simulink model "dynamic_block"  (R2023b)
settings: Solver=VariableStepAuto  StartTime=0.0  StopTime=10.0  RelTol=1e-3
libraries: matrix_library x1, aerolibutil x1
settings Model: Creator=aryam  LastModifiedBy=aryam

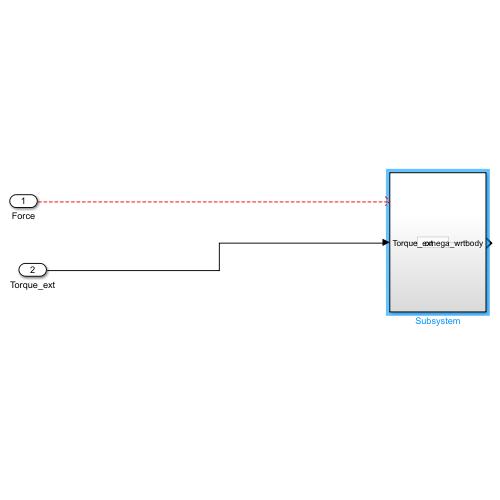
[thumbnail: Simulink's stored preview of the top-level diagram]
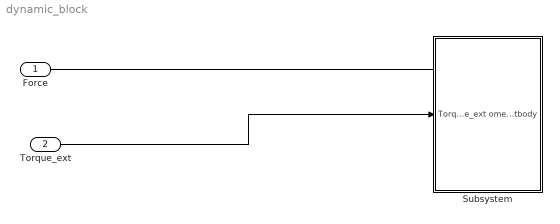
== system dynamic_block ==
  Force : Inport
  Torque_ext : Inport  Port=2  PortDimensions=3
  Subsystem : Subsystem
  wires:
  Force/1 -> ?
  Torque_ext/1 -> Subsystem/1(Torque_ext)

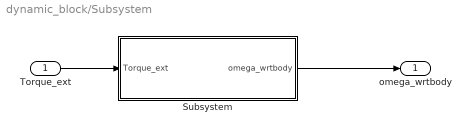
== system dynamic_block/Subsystem ==
  Torque_ext : Inport  PortDimensions=3
  Subsystem : Subsystem
  omega_wrtbody : Outport
  wires:
  Torque_ext/1 -> Subsystem/1(Torque_ext)
  Subsystem/1(omega_wrtbody) -> omega_wrtbody/1

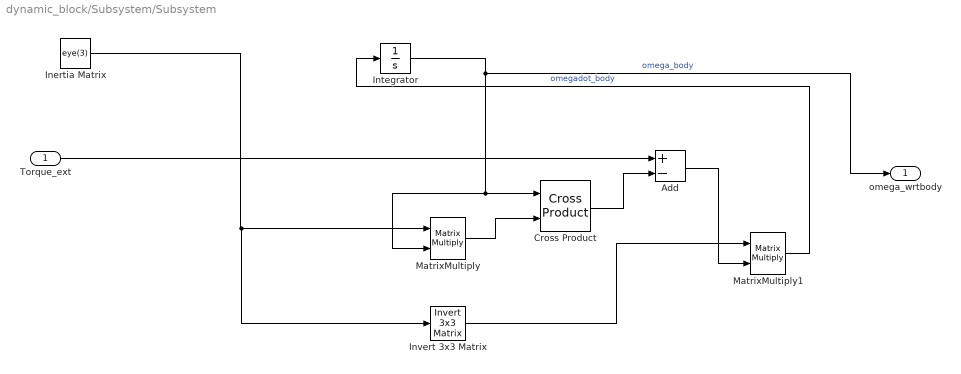
== system dynamic_block/Subsystem/Subsystem ==
  Torque_ext : Inport  PortDimensions=3
  Add : Sum  Inputs=+-
  Cross Product : matrix_library/Cross Product
  Inertia Matrix : Constant  Value=eye(3)
  Integrator : Integrator  InitialCondition=[0, 0, 0]
  Invert 3x3 Matrix : aerolibutil/Invert  3x3 Matrix
  MatrixMultiply : Product  Multiplication=Matrix(*)
  MatrixMultiply1 : Product  Multiplication=Matrix(*)
  omega_wrtbody : Outport
  wires:
  Add/1 -> MatrixMultiply1/2
  Inertia Matrix/1 -> Invert 3x3 Matrix/1, MatrixMultiply/1
  Integrator/1 -> omega_wrtbody/1, Cross Product/1, MatrixMultiply/2  "omega_body"
  MatrixMultiply1/1 -> Integrator/1  "omegadot_body"
  MatrixMultiply/1 -> Cross Product/2
  Invert 3x3 Matrix/1 -> MatrixMultiply1/1
  Cross Product/1 -> Add/2
  Torque_ext/1 -> Add/1
